simulink model "Exemplu_figura18"  (R2016a)
settings: Solver=VariableStepDiscrete  StartTime=0.0  StopTime=30  RelTol=1e-3
undefined symbols (not defined in the file): entity, f, g, m
settings Model: Creator=Cristina  LastModifiedBy=Cristina

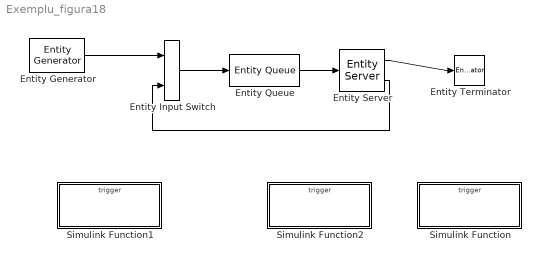
== system Exemplu_figura18 ==
  Entity Input Switch : EntityInputSwitch  InputPortMessageModes=m,m  OutputPortMessageModes=m
  Entity Generator : EntityGenerator  OutputPortMessageModes=m  GenerateAction=|  ExitAction=g(entity.Priority);  AttributeName=Priority|ServiceTime|Preempted  AttributeInitialValue=1|1|0  EntityType=Structured  EntityTypeName=Entity
      | if rand < 0.3
      |     entity.Priority = 1;
      |     entity.ServiceTime = 0.9;
      | else
      |     entity.Priority = 2;
      |     entity.ServiceTime = 1.1;
      | end
  Entity Queue : EntityQueue  InputPortMessageModes=m  OutputPortMessageModes=m  QueueType=Priority  PrioritySource=Priority
      settings: OutputPortMap=o5
  Entity Server : EntityServer  InputPortMessageModes=m  OutputPortMessageModes=m,m  Capacity=1  PreemptAction=|  PermitPreemptionBasedOnAttribute=on  SortingAttributeName=Priority  ResidualTimeAttributeName=ServiceTime
      | entity.Preempted = entity.Preempted + 1;
      | p(entity.ServiceTime);
      settings: OutputPortMap=o9,o10
  Entity Terminator : EntityTerminator  InputPortMessageModes=m  EntryAction=f(entity.Preempted);
  Simulink Function : Subsystem  TreatAsAtomicUnit=on
  Simulink Function1 : Subsystem  TreatAsAtomicUnit=on
  Simulink Function2 : Subsystem  TreatAsAtomicUnit=on
  wires:
  Entity Generator/1 -> Entity Input Switch/1
  Entity Input Switch/1 -> Entity Queue/1
  Entity Queue/1 -> Entity Server/1
  Entity Server/1 -> Entity Terminator/1
  Entity Server/2 -> Entity Input Switch/2

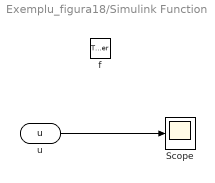
== system Exemplu_figura18/Simulink Function ==
  f : TriggerPort  TriggerType=function-call  IsSimulinkFunction=on  FunctionName=f  VariantControl=Variant
  Scope : Scope
  u : ArgIn  DisableCoverage=on  ArgumentName=u
  wires:
  u/1 -> Scope/1

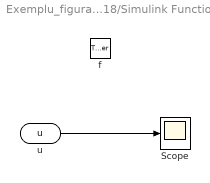
== system Exemplu_figura18/Simulink Function1 ==
  f : TriggerPort  TriggerType=function-call  IsSimulinkFunction=on  FunctionName=g  VariantControl=Variant
  Scope : Scope
  u : ArgIn  DisableCoverage=on  ArgumentName=u
  wires:
  u/1 -> Scope/1

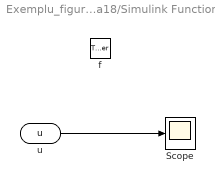
== system Exemplu_figura18/Simulink Function2 ==
  f : TriggerPort  TriggerType=function-call  IsSimulinkFunction=on  FunctionName=p  VariantControl=Variant
  Scope : Scope
  u : ArgIn  DisableCoverage=on  ArgumentName=u
  wires:
  u/1 -> Scope/1
